simulink model "sm_ratchet_lifter"  (R2020b)
settings: Solver=daessc  StartTime=0.0  StopTime=20  MaxStep=1e-3  RelTol=1e-3  EnableMultiTasking=on
model workspace: external: MATLAB File sm_ratchet_lifter_parameters.m (data not in the file)
undefined symbols (not defined in the file or in its folder): climber, contact, cyl1, cyl10, cyl11, cyl12, cyl13, cyl14, cyl15, cyl2, cyl3, cyl4, cyl5, cyl6, cyl7, cyl8, cyl9, hook, init, LeftHorizCyl, LeftSlantCyl, load, rack, RightHorizCyl, RightSlantCyl, traveler, X, Y, Z
libraries: sm_lib x223, nesl_utility x4
(part 2 of 5)

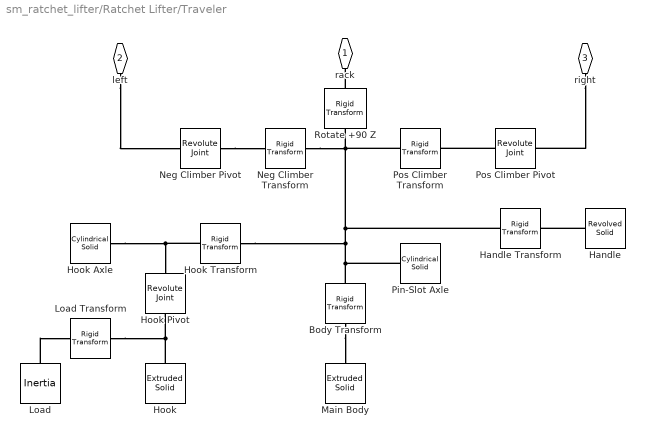
== system sm_ratchet_lifter/Ratchet Lifter/Traveler ==
  Body Transform : sm_lib/Frames and Transforms/Rigid Transform  TranslationMethod=None  TranslationStandardOffset=0  TranslationLengthUnit=m  TranslationStandardAxis=+Z  TranslationCartesianOffset=[0 0 0]  TranslationROffset=0  TranslationROffsetUnits=m  TranslationZOffset=0  TranslationZOffsetUnits=m  TranslationThetaOffset=0  TranslationThetaOffsetUnits=deg  RotationMethod=AlignedAxes  RotationAngleUnits=deg  RotationStandardAxis=+Z  RotationAngle=0.0  RotationArbitraryAxis=[0 0 1]  FollAlignAxisA=+Z  BaseAlignAxisA=+Y  FollAlignAxisB=+X  BaseAlignAxisB=-Z  RotationSequenceAxes=FollowerAxes  RotationSequence=XYX  RotationSequenceAngles=[0 0 0]  RotationSequenceAnglesUnits=deg  RotationMatrix=[1 0 0; 0 1 0; 0 0 1]
      settings: SourceProductName=Multibody
  Handle : sm_lib/Body Elements/Revolved Solid  GraphicAmbientColor=[0.15 0.15 0.15 1.0]  BasedOnType=Density  CenterOfMass=[0 0 0]  CenterOfMassUnits=m  GraphicDiffuseColor=color.handle_color  ExportConvexHullGeometry=off  Density=1000  DensityUnits=kg/m^3  DoExposeReferenceFrame=on  GraphicEmissiveColor=[0.0 0.0 0.0 1.0]  ExportEntireGeometry=off  SerializedFrames=<Frames/>  MarkerShape=Sphere  MarkerSize=10  GraphicType=FromGeometry  InertiaType=CalculateFromGeometry  Mass=1  MassUnits=kg  MomentsOfInertia=[1 1 1]  MomentsOfInertiaUnits=kg*m^2  GraphicOpacity=1.0  ProductsOfInertia=[0 0 0]  ProductsOfInertiaUnits=kg*m^2  RevolutionCrossSection=traveler.handle_xsect  RevolutionCrossSectionUnits=cm  RevolutionAngle=180  RevolutionAngleUnits=deg  RevolutionExtent=Full  GraphicShininess=75  GraphicSpecularColor=[0.5 0.5 0.5 1.0]  GraphicVisPropType=SimpleVisualProperties
      settings: SourceProductName=Multibody
  Handle Transform : sm_lib/Frames and Transforms/Rigid Transform  TranslationMethod=StandardAxis  TranslationStandardOffset=traveler.length / 2  TranslationLengthUnit=cm  TranslationStandardAxis=+X  TranslationCartesianOffset=[0 0 0]  TranslationROffset=0  TranslationROffsetUnits=m  TranslationZOffset=0  TranslationZOffsetUnits=m  TranslationThetaOffset=0  TranslationThetaOffsetUnits=deg  RotationMethod=AlignedAxes  RotationAngleUnits=deg  RotationStandardAxis=+Z  RotationAngle=0.0  RotationArbitraryAxis=[0 0 1]  FollAlignAxisA=+Z  BaseAlignAxisA=+X  FollAlignAxisB=+X  BaseAlignAxisB=+Z  RotationSequenceAxes=FollowerAxes  RotationSequence=XYX  RotationSequenceAngles=[0 0 0]  RotationSequenceAnglesUnits=deg  RotationMatrix=[1 0 0; 0 1 0; 0 0 1]
      settings: SourceProductName=Multibody
  Hook : sm_lib/Body Elements/Extruded Solid  GraphicAmbientColor=[0.15 0.15 0.15 1.0]  BasedOnType=Density  CenterOfMass=[0 0 0]  CenterOfMassUnits=m  GraphicDiffuseColor=color.hook_color  ExportConvexHullGeometry=off  ExtrusionCrossSection=hook.xsect  ExtrusionCrossSectionUnits=cm  Density=1000  DensityUnits=kg/m^3  DoExposeReferenceFrame=on  GraphicEmissiveColor=[0.0 0.0 0.0 1.0]  ExportEntireGeometry=off  ExtrusionLength=hook.thick  ExtrusionLengthUnits=cm  ExtrusionType=General  SerializedFrames=<Frames/>  MarkerShape=Sphere  MarkerSize=10  GraphicType=FromGeometry  InertiaType=CalculateFromGeometry  Mass=1  MassUnits=kg  MomentsOfInertia=[1 1 1]  MomentsOfInertiaUnits=kg*m^2  PolygonNumSides=3  GraphicOpacity=1.0  PolygonOuterRadius=1  PolygonOuterRadiusUnits=m  ProductsOfInertia=[0 0 0]  ProductsOfInertiaUnits=kg*m^2  GraphicShininess=75  GraphicSpecularColor=[0.5 0.5 0.5 1.0]  GraphicVisPropType=SimpleVisualProperties
      settings: SourceProductName=Multibody
  Hook Transform : sm_lib/Frames and Transforms/Rigid Transform  TranslationMethod=StandardAxis  TranslationStandardOffset=-traveler.length/2 + traveler.end_hole_length/2  TranslationLengthUnit=cm  TranslationStandardAxis=-X  TranslationCartesianOffset=[0 0 0]  TranslationROffset=0  TranslationROffsetUnits=m  TranslationZOffset=0  TranslationZOffsetUnits=m  TranslationThetaOffset=0  TranslationThetaOffsetUnits=deg  RotationMethod=None  RotationAngleUnits=deg  RotationStandardAxis=+Z  RotationAngle=0.0  RotationArbitraryAxis=[0 0 1]  FollAlignAxisA=+X  BaseAlignAxisA=+Y  FollAlignAxisB=+Y  BaseAlignAxisB=+Z  RotationSequenceAxes=FollowerAxes  RotationSequence=XYX  RotationSequenceAngles=[0 0 0]  RotationSequenceAnglesUnits=deg  RotationMatrix=[1 0 0; 0 1 0; 0 0 1]
      settings: SourceProductName=Multibody
  Hook Axle : sm_lib/Body Elements/Cylindrical Solid  GraphicAmbientColor=[0.15 0.15 0.15 1.0]  BasedOnType=Density  CenterOfMass=[0 0 0]  CenterOfMassUnits=m  GraphicDiffuseColor=color.traveler_axle_color  CylinderLength=traveler.axle_length  CylinderLengthUnits=cm  CylinderRadius=traveler.hook_axle_rad  CylinderRadiusUnits=cm  Density=1000  DensityUnits=kg/m^3  DoExposeReferenceFrame=on  GraphicEmissiveColor=[0.0 0.0 0.0 1.0]  ExportEntireGeometry=off  SerializedFrames=<Frames/>  MarkerShape=Sphere  MarkerSize=10  GraphicType=FromGeometry  InertiaType=CalculateFromGeometry  Mass=1  MassUnits=kg  MomentsOfInertia=[1 1 1]  MomentsOfInertiaUnits=kg*m^2  GraphicOpacity=1.0  ProductsOfInertia=[0 0 0]  ProductsOfInertiaUnits=kg*m^2  GraphicShininess=75  GraphicSpecularColor=[0.5 0.5 0.5 1.0]  GraphicVisPropType=SimpleVisualProperties
      settings: SourceProductName=Multibody
  Hook Pivot : sm_lib/Joints/Revolute Joint  JointMode=Normal  SenseConstraintForce=off  SenseConstraintForceX=off  SenseConstraintForceY=off  SenseConstraintForceZ=off  SenseConstraintTorque=off  SenseConstraintTorqueX=off  SenseConstraintTorqueY=off  SenseConstraintTorqueZ=off  SenseTotalForce=off  SenseTotalForceX=off  SenseTotalForceY=off  SenseTotalForceZ=off  SenseTotalTorque=off  SenseTotalTorqueX=off  SenseTotalTorqueY=off  SenseTotalTorqueZ=off  CompositeWrenchDir=FollowerOnBase  CompositeWrenchFrame=BaseFrame  EquilibriumPosition=0  EquilibriumPositionUnits=deg  SpringStiffness=0  SpringStiffnessUnits=N*m/deg  DampingCoefficient=0  DampingCoefficientUnits=N*m/(deg/s)  TorqueActuationMode=NoTorque  MotionActuationMode=ComputedMotion  SensePosition=off  SenseVelocity=off  SenseAcceleration=off  SenseTorqueForce=off  SenseLowerLimitTorqueForce=off  SenseUpperLimitTorqueForce=off  LowerLimitSpecify=off  LowerLimitBound=-90  LowerLimitBoundUnits=deg  LowerLimitStiffness=1e4  LowerLimitStiffnessUnits=N*m/deg  LowerLimitDamping=10  LowerLimitDampingUnits=N*m/(deg/s)  LowerLimitTransitionRegionWidth=0.1  LowerLimitTransitionRegionWidthUnits=deg  UpperLimitSpecify=off  UpperLimitBound=90  UpperLimitBoundUnits=deg  UpperLimitStiffness=1e4  UpperLimitStiffnessUnits=N*m/deg  UpperLimitDamping=10  UpperLimitDampingUnits=N*m/(deg/s)  UpperLimitTransitionRegionWidth=0.1  UpperLimitTransitionRegionWidthUnits=deg  PositionTargetSpecify=off  PositionTargetPriority=High  PositionTargetValue=0  PositionTargetValueUnits=deg  VelocityTargetSpecify=off  VelocityTargetPriority=High  VelocityTargetValue=0  VelocityTargetValueUnits=deg/s
      settings: SourceProductName=Multibody
  Load : sm_lib/Body Elements/Inertia  InertiaType=PointMass  Mass=load.mass  MassUnits=g  CenterOfMass=[0 0 0]  CenterOfMassUnits=m  MomentsOfInertia=[1 1 1]  MomentsOfInertiaUnits=kg*m^2  ProductsOfInertia=[0 0 0]  ProductsOfInertiaUnits=kg*m^2  GraphicType=None  MarkerShape=Inertia  MarkerSize=20  GraphicVisPropType=SimpleVisualProperties  GraphicDiffuseColor=[0.5 0.5 0.5]  GraphicSpecularColor=[0.5 0.5 0.5 1.0]  GraphicAmbientColor=[0.15 0.15 0.15 1.0]  GraphicEmissiveColor=[0.0 0.0 0.0 1.0]  GraphicShininess=75  GraphicOpacity=1.0
      settings: SourceProductName=Multibody
  Load Transform : sm_lib/Frames and Transforms/Rigid Transform  TranslationMethod=Cartesian  TranslationStandardOffset=0  TranslationLengthUnit=cm  TranslationStandardAxis=+Z  TranslationCartesianOffset=[hook.offset, 0] + load.dist * [0 -1 0]  TranslationROffset=0  TranslationROffsetUnits=m  TranslationZOffset=0  TranslationZOffsetUnits=m  TranslationThetaOffset=0  TranslationThetaOffsetUnits=deg  RotationMethod=None  RotationAngleUnits=deg  RotationStandardAxis=+Z  RotationAngle=0.0  RotationArbitraryAxis=[0 0 1]  FollAlignAxisA=+X  BaseAlignAxisA=+Y  FollAlignAxisB=+Y  BaseAlignAxisB=+Z  RotationSequenceAxes=FollowerAxes  RotationSequence=XYX  RotationSequenceAngles=[0 0 0]  RotationSequenceAnglesUnits=deg  RotationMatrix=[1 0 0; 0 1 0; 0 0 1]
      settings: SourceProductName=Multibody
  Main Body : sm_lib/Body Elements/Extruded Solid  GraphicAmbientColor=[0.15 0.15 0.15 1.0]  BasedOnType=Density  CenterOfMass=[0 0 0]  CenterOfMassUnits=m  GraphicDiffuseColor=color.traveler_color  ExportConvexHullGeometry=off  ExtrusionCrossSection=traveler.xsect  ExtrusionCrossSectionUnits=cm  Density=1000  DensityUnits=kg/m^3  DoExposeReferenceFrame=on  GraphicEmissiveColor=[0.0 0.0 0.0 1.0]  ExportEntireGeometry=off  ExtrusionLength=traveler.width  ExtrusionLengthUnits=cm  ExtrusionType=General  SerializedFrames=<Frames/>  MarkerShape=Sphere  MarkerSize=10  GraphicType=FromGeometry  InertiaType=CalculateFromGeometry  Mass=1  MassUnits=kg  MomentsOfInertia=[1 1 1]  MomentsOfInertiaUnits=kg*m^2  PolygonNumSides=3  GraphicOpacity=1.0  PolygonOuterRadius=1  PolygonOuterRadiusUnits=m  ProductsOfInertia=[0 0 0]  ProductsOfInertiaUnits=kg*m^2  GraphicShininess=75  GraphicSpecularColor=[0.5 0.5 0.5 1.0]  GraphicVisPropType=SimpleVisualProperties
      settings: SourceProductName=Multibody
  Neg Climber Pivot : sm_lib/Joints/Revolute Joint  JointMode=Normal  SenseConstraintForce=off  SenseConstraintForceX=off  SenseConstraintForceY=off  SenseConstraintForceZ=off  SenseConstraintTorque=off  SenseConstraintTorqueX=off  SenseConstraintTorqueY=off  SenseConstraintTorqueZ=off  SenseTotalForce=off  SenseTotalForceX=off  SenseTotalForceY=off  SenseTotalForceZ=off  SenseTotalTorque=off  SenseTotalTorqueX=off  SenseTotalTorqueY=off  SenseTotalTorqueZ=off  CompositeWrenchDir=FollowerOnBase  CompositeWrenchFrame=BaseFrame  EquilibriumPosition=0  EquilibriumPositionUnits=deg  SpringStiffness=0  SpringStiffnessUnits=N*m/deg  DampingCoefficient=0  DampingCoefficientUnits=N*m/(deg/s)  TorqueActuationMode=NoTorque  MotionActuationMode=ComputedMotion  SensePosition=off  SenseVelocity=off  SenseAcceleration=off  SenseTorqueForce=off  SenseLowerLimitTorqueForce=off  SenseUpperLimitTorqueForce=off  LowerLimitSpecify=off  LowerLimitBound=-90  LowerLimitBoundUnits=deg  LowerLimitStiffness=1e4  LowerLimitStiffnessUnits=N*m/deg  LowerLimitDamping=10  LowerLimitDampingUnits=N*m/(deg/s)  LowerLimitTransitionRegionWidth=0.1  LowerLimitTransitionRegionWidthUnits=deg  UpperLimitSpecify=off  UpperLimitBound=90  UpperLimitBoundUnits=deg  UpperLimitStiffness=1e4  UpperLimitStiffnessUnits=N*m/deg  UpperLimitDamping=10  UpperLimitDampingUnits=N*m/(deg/s)  UpperLimitTransitionRegionWidth=0.1  UpperLimitTransitionRegionWidthUnits=deg  PositionTargetSpecify=on  PositionTargetPriority=High  PositionTargetValue=pi/2 + init.climber_angle  PositionTargetValueUnits=rad  VelocityTargetSpecify=off  VelocityTargetPriority=High  VelocityTargetValue=0  VelocityTargetValueUnits=deg/s
      settings: SourceProductName=Multibody
  Neg Climber Transform : sm_lib/Frames and Transforms/Rigid Transform  TranslationMethod=StandardAxis  TranslationStandardOffset=traveler.climber_offset  TranslationLengthUnit=cm  TranslationStandardAxis=-X  TranslationCartesianOffset=[0 0 0]  TranslationROffset=0  TranslationROffsetUnits=m  TranslationZOffset=0  TranslationZOffsetUnits=m  TranslationThetaOffset=0  TranslationThetaOffsetUnits=deg  RotationMethod=None  RotationAngleUnits=deg  RotationStandardAxis=+Z  RotationAngle=0.0  RotationArbitraryAxis=[0 0 1]  FollAlignAxisA=+X  BaseAlignAxisA=+Y  FollAlignAxisB=+Y  BaseAlignAxisB=+Z  RotationSequenceAxes=FollowerAxes  RotationSequence=XYX  RotationSequenceAngles=[0 0 0]  RotationSequenceAnglesUnits=deg  RotationMatrix=[1 0 0; 0 1 0; 0 0 1]
      settings: SourceProductName=Multibody
  Pin-Slot Axle : sm_lib/Body Elements/Cylindrical Solid  GraphicAmbientColor=[0.15 0.15 0.15 1.0]  BasedOnType=Density  CenterOfMass=[0 0 0]  CenterOfMassUnits=m  GraphicDiffuseColor=color.traveler_axle_color  CylinderLength=traveler.axle_length  CylinderLengthUnits=cm  CylinderRadius=traveler.slot_half_width  CylinderRadiusUnits=cm  Density=1000  DensityUnits=kg/m^3  DoExposeReferenceFrame=on  GraphicEmissiveColor=[0.0 0.0 0.0 1.0]  ExportEntireGeometry=off  SerializedFrames=<Frames/>  MarkerShape=Sphere  MarkerSize=10  GraphicType=FromGeometry  InertiaType=CalculateFromGeometry  Mass=1  MassUnits=kg  MomentsOfInertia=[1 1 1]  MomentsOfInertiaUnits=kg*m^2  GraphicOpacity=1.0  ProductsOfInertia=[0 0 0]  ProductsOfInertiaUnits=kg*m^2  GraphicShininess=75  GraphicSpecularColor=[0.5 0.5 0.5 1.0]  GraphicVisPropType=SimpleVisualProperties
      settings: SourceProductName=Multibody
  Pos Climber Pivot : sm_lib/Joints/Revolute Joint  JointMode=Normal  SenseConstraintForce=off  SenseConstraintForceX=off  SenseConstraintForceY=off  SenseConstraintForceZ=off  SenseConstraintTorque=off  SenseConstraintTorqueX=off  SenseConstraintTorqueY=off  SenseConstraintTorqueZ=off  SenseTotalForce=off  SenseTotalForceX=off  SenseTotalForceY=off  SenseTotalForceZ=off  SenseTotalTorque=off  SenseTotalTorqueX=off  SenseTotalTorqueY=off  SenseTotalTorqueZ=off  CompositeWrenchDir=FollowerOnBase  CompositeWrenchFrame=BaseFrame  EquilibriumPosition=0  EquilibriumPositionUnits=deg  SpringStiffness=0  SpringStiffnessUnits=N*m/deg  DampingCoefficient=0  DampingCoefficientUnits=N*m/(deg/s)  TorqueActuationMode=NoTorque  MotionActuationMode=ComputedMotion  SensePosition=off  SenseVelocity=off  SenseAcceleration=off  SenseTorqueForce=off  SenseLowerLimitTorqueForce=off  SenseUpperLimitTorqueForce=off  LowerLimitSpecify=off  LowerLimitBound=-90  LowerLimitBoundUnits=deg  LowerLimitStiffness=1e4  LowerLimitStiffnessUnits=N*m/deg  LowerLimitDamping=10  LowerLimitDampingUnits=N*m/(deg/s)  LowerLimitTransitionRegionWidth=0.1  LowerLimitTransitionRegionWidthUnits=deg  UpperLimitSpecify=off  UpperLimitBound=90  UpperLimitBoundUnits=deg  UpperLimitStiffness=1e4  UpperLimitStiffnessUnits=N*m/deg  UpperLimitDamping=10  UpperLimitDampingUnits=N*m/(deg/s)  UpperLimitTransitionRegionWidth=0.1  UpperLimitTransitionRegionWidthUnits=deg  PositionTargetSpecify=on  PositionTargetPriority=High  PositionTargetValue=pi/2 - init.climber_angle  PositionTargetValueUnits=rad  VelocityTargetSpecify=off  VelocityTargetPriority=High  VelocityTargetValue=0  VelocityTargetValueUnits=deg/s
      settings: SourceProductName=Multibody
  Pos Climber Transform : sm_lib/Frames and Transforms/Rigid Transform  TranslationMethod=StandardAxis  TranslationStandardOffset=traveler.climber_offset  TranslationLengthUnit=cm  TranslationStandardAxis=+X  TranslationCartesianOffset=[0 0 0]  TranslationROffset=0  TranslationROffsetUnits=m  TranslationZOffset=0  TranslationZOffsetUnits=m  TranslationThetaOffset=0  TranslationThetaOffsetUnits=deg  RotationMethod=None  RotationAngleUnits=deg  RotationStandardAxis=+Z  RotationAngle=0.0  RotationArbitraryAxis=[0 0 1]  FollAlignAxisA=+X  BaseAlignAxisA=+Y  FollAlignAxisB=+Y  BaseAlignAxisB=+Z  RotationSequenceAxes=FollowerAxes  RotationSequence=XYX  RotationSequenceAngles=[0 0 0]  RotationSequenceAnglesUnits=deg  RotationMatrix=[1 0 0; 0 1 0; 0 0 1]
      settings: SourceProductName=Multibody
  Rotate +90 Z : sm_lib/Frames and Transforms/Rigid Transform  TranslationMethod=None  TranslationStandardOffset=0  TranslationLengthUnit=m  TranslationStandardAxis=+Z  TranslationCartesianOffset=[0 0 0]  TranslationROffset=0  TranslationROffsetUnits=m  TranslationZOffset=0  TranslationZOffsetUnits=m  TranslationThetaOffset=0  TranslationThetaOffsetUnits=deg  RotationMethod=StandardAxis  RotationAngleUnits=deg  RotationStandardAxis=+Z  RotationAngle=90  RotationArbitraryAxis=[0 0 1]  FollAlignAxisA=+X  BaseAlignAxisA=+Y  FollAlignAxisB=+Y  BaseAlignAxisB=+Z  RotationSequenceAxes=FollowerAxes  RotationSequence=XYX  RotationSequenceAngles=[0 0 0]  RotationSequenceAnglesUnits=deg  RotationMatrix=[1 0 0; 0 1 0; 0 0 1]
      settings: SourceProductName=Multibody
  rack : PMIOPort  Side=Left
  left : PMIOPort  Port=2  Side=Left
  right : PMIOPort  Port=3  Side=Right
  connections:
  Pin-Slot Axle/RConn1 -- Hook Transform/RConn1 -- Handle Transform/LConn1 -- Pos Climber Transform/LConn1 -- Rotate +90 Z/LConn1 -- Neg Climber Transform/LConn1 -- Body Transform/LConn1
  Pos Climber Pivot/LConn1 -- Pos Climber Transform/RConn1
  left/RConn1 -- Neg Climber Pivot/RConn1
  right/RConn1 -- Pos Climber Pivot/RConn1
  Rotate +90 Z/RConn1 -- rack/RConn1
  Neg Climber Pivot/LConn1 -- Neg Climber Transform/RConn1
  Handle/RConn1 -- Handle Transform/RConn1
  Body Transform/RConn1 -- Main Body/RConn1
  Hook Transform/LConn1 -- Hook Axle/RConn1 -- Hook Pivot/LConn1
  Hook/RConn1 -- Load Transform/LConn1 -- Hook Pivot/RConn1
  Load/RConn1 -- Load Transform/RConn1

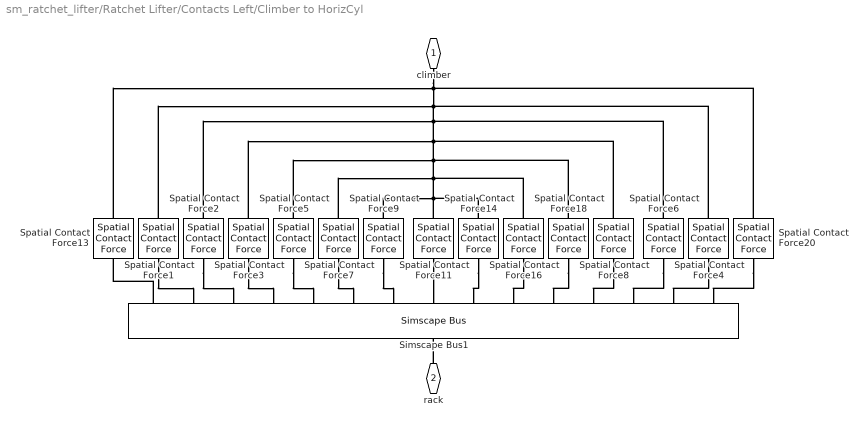
== system sm_ratchet_lifter/Ratchet Lifter/Contacts Left/Climber to HorizCyl ==
  Simscape Bus1 : SimscapeBus  HierarchyStrings=cyl15;cyl14;cyl13;cyl12;cyl11;cyl10;cyl9;cyl8;cyl7;cyl6;cyl5;cyl4;cyl3;cyl2;cyl1
  Spatial Contact Force{1..9,11,13..14,16,18,20} (15 alike) : sm_lib/Forces and Torques/Spatial Contact Force  CoefficientOfDynamicFriction=muk  CoefficientOfStaticFriction=mus  NormalDamping=b  NormalDampingUnits=N/(m/s)  NormalStiffness=k  NormalStiffnessUnits=N/m  FrictionalCriticalVelocity=cv  FrictionalCriticalVelocityUnits=cm/s  ZeroCrossDetectContactStartAndEnd=off  SenseFrictionalForceMagnitude=off  SenseNormalForceMagnitude=off  SenseSeparationDistance=off  NormalTransitionRegionWidth=tau  NormalTransitionRegionWidthUnits=mm  FrictionType=SmoothStickSlip
      settings: SourceProductName=Multibody
  climber : PMIOPort  Side=Right
  rack : PMIOPort  Port=2  Side=Left
  connections:
  Spatial Contact Force13/RConn1 -- Spatial Contact Force20/RConn1 -- Spatial Contact Force4/RConn1 -- Spatial Contact Force1/RConn1 -- Spatial Contact Force6/RConn1 -- Spatial Contact Force2/RConn1 -- Spatial Contact Force8/RConn1 -- Spatial Contact Force3/RConn1 -- Spatial Contact Force18/RConn1 -- Spatial Contact Force5/RConn1 -- Spatial Contact Force16/RConn1 -- Spatial Contact Force7/RConn1 -- Spatial Contact Force14/RConn1 -- Spatial Contact Force11/RConn1 -- Spatial Contact Force9/RConn1 -- climber/RConn1
  Spatial Contact Force11/LConn1 -- Simscape Bus1/LConn8
  Spatial Contact Force8/LConn1 -- Simscape Bus1/LConn12
  Spatial Contact Force7/LConn1 -- Simscape Bus1/LConn6
  Simscape Bus1/LConn1 -- Spatial Contact Force13/LConn1
  Spatial Contact Force5/LConn1 -- Simscape Bus1/LConn5
  Spatial Contact Force2/LConn1 -- Simscape Bus1/LConn3
  Spatial Contact Force18/LConn1 -- Simscape Bus1/LConn11
  Spatial Contact Force9/LConn1 -- Simscape Bus1/LConn7
  Spatial Contact Force14/LConn1 -- Simscape Bus1/LConn9
  Spatial Contact Force1/LConn1 -- Simscape Bus1/LConn2
  rack/RConn1 -- Simscape Bus1/RConn1
  Spatial Contact Force16/LConn1 -- Simscape Bus1/LConn10
  Spatial Contact Force20/LConn1 -- Simscape Bus1/LConn15
  Spatial Contact Force4/LConn1 -- Simscape Bus1/LConn14
  Spatial Contact Force3/LConn1 -- Simscape Bus1/LConn4
  Spatial Contact Force6/LConn1 -- Simscape Bus1/LConn13

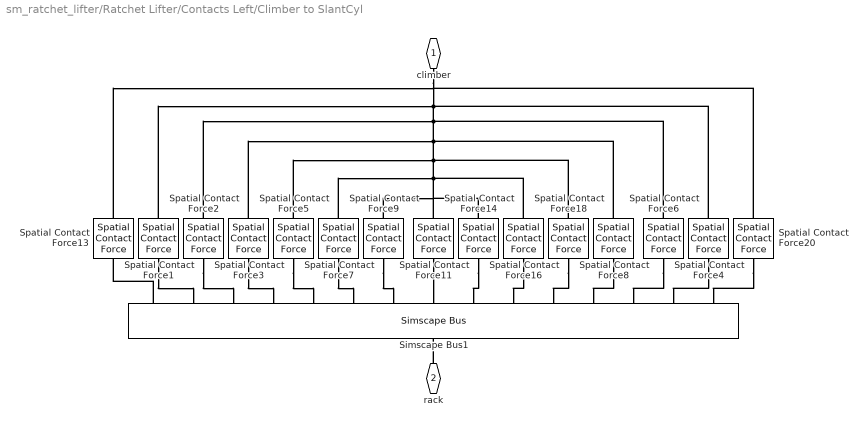
== system sm_ratchet_lifter/Ratchet Lifter/Contacts Left/Climber to SlantCyl ==
  Simscape Bus1 : SimscapeBus  HierarchyStrings=cyl15;cyl14;cyl13;cyl12;cyl11;cyl10;cyl9;cyl8;cyl7;cyl6;cyl5;cyl4;cyl3;cyl2;cyl1
  Spatial Contact Force{1..9,11,13..14,16,18,20} (15 alike) : sm_lib/Forces and Torques/Spatial Contact Force  CoefficientOfDynamicFriction=muk  CoefficientOfStaticFriction=mus  NormalDamping=b  NormalDampingUnits=N/(m/s)  NormalStiffness=k  NormalStiffnessUnits=N/m  FrictionalCriticalVelocity=cv  FrictionalCriticalVelocityUnits=cm/s  ZeroCrossDetectContactStartAndEnd=off  SenseFrictionalForceMagnitude=off  SenseNormalForceMagnitude=off  SenseSeparationDistance=off  NormalTransitionRegionWidth=tau  NormalTransitionRegionWidthUnits=mm  FrictionType=SmoothStickSlip
      settings: SourceProductName=Multibody
  climber : PMIOPort  Side=Right
  rack : PMIOPort  Port=2  Side=Left
  connections:
  Spatial Contact Force14/RConn1 -- Spatial Contact Force11/RConn1 -- Spatial Contact Force9/RConn1 -- Spatial Contact Force16/RConn1 -- Spatial Contact Force7/RConn1 -- Spatial Contact Force18/RConn1 -- Spatial Contact Force5/RConn1 -- Spatial Contact Force8/RConn1 -- Spatial Contact Force3/RConn1 -- Spatial Contact Force6/RConn1 -- Spatial Contact Force2/RConn1 -- Spatial Contact Force4/RConn1 -- Spatial Contact Force1/RConn1 -- Spatial Contact Force20/RConn1 -- climber/RConn1 -- Spatial Contact Force13/RConn1
  rack/RConn1 -- Simscape Bus1/RConn1
  Spatial Contact Force20/LConn1 -- Simscape Bus1/LConn15
  Spatial Contact Force4/LConn1 -- Simscape Bus1/LConn14
  Spatial Contact Force6/LConn1 -- Simscape Bus1/LConn13
  Spatial Contact Force8/LConn1 -- Simscape Bus1/LConn12
  Spatial Contact Force18/LConn1 -- Simscape Bus1/LConn11
  Spatial Contact Force16/LConn1 -- Simscape Bus1/LConn10
  Spatial Contact Force14/LConn1 -- Simscape Bus1/LConn9
  Spatial Contact Force11/LConn1 -- Simscape Bus1/LConn8
  Spatial Contact Force9/LConn1 -- Simscape Bus1/LConn7
  Spatial Contact Force7/LConn1 -- Simscape Bus1/LConn6
  Spatial Contact Force5/LConn1 -- Simscape Bus1/LConn5
  Spatial Contact Force3/LConn1 -- Simscape Bus1/LConn4
  Spatial Contact Force2/LConn1 -- Simscape Bus1/LConn3
  Spatial Contact Force1/LConn1 -- Simscape Bus1/LConn2
  Simscape Bus1/LConn1 -- Spatial Contact Force13/LConn1

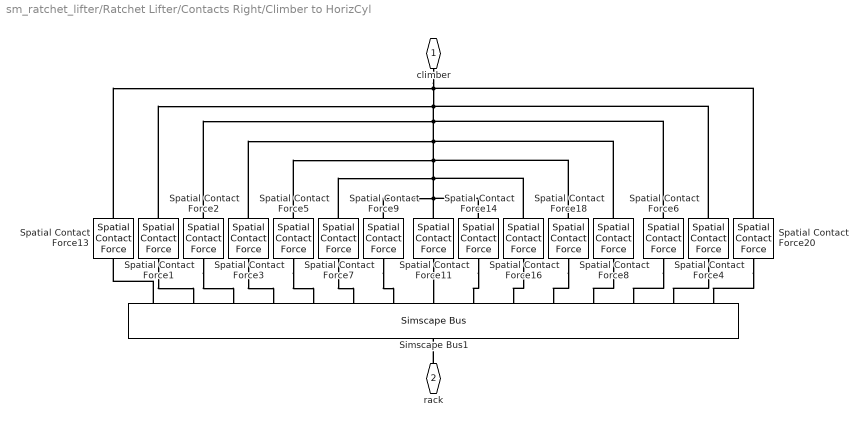
== system sm_ratchet_lifter/Ratchet Lifter/Contacts Right/Climber to HorizCyl ==
  Simscape Bus1 : SimscapeBus  HierarchyStrings=cyl15;cyl14;cyl13;cyl12;cyl11;cyl10;cyl9;cyl8;cyl7;cyl6;cyl5;cyl4;cyl3;cyl2;cyl1
  Spatial Contact Force{1..9,11,13..14,16,18,20} (15 alike) : sm_lib/Forces and Torques/Spatial Contact Force  CoefficientOfDynamicFriction=muk  CoefficientOfStaticFriction=mus  NormalDamping=b  NormalDampingUnits=N/(m/s)  NormalStiffness=k  NormalStiffnessUnits=N/m  FrictionalCriticalVelocity=cv  FrictionalCriticalVelocityUnits=cm/s  ZeroCrossDetectContactStartAndEnd=off  SenseFrictionalForceMagnitude=off  SenseNormalForceMagnitude=off  SenseSeparationDistance=off  NormalTransitionRegionWidth=tau  NormalTransitionRegionWidthUnits=mm  FrictionType=SmoothStickSlip
      settings: SourceProductName=Multibody
  climber : PMIOPort  Side=Right
  rack : PMIOPort  Port=2  Side=Left
  connections:
  Spatial Contact Force13/RConn1 -- Spatial Contact Force20/RConn1 -- Spatial Contact Force4/RConn1 -- Spatial Contact Force1/RConn1 -- Spatial Contact Force6/RConn1 -- Spatial Contact Force2/RConn1 -- Spatial Contact Force8/RConn1 -- Spatial Contact Force3/RConn1 -- Spatial Contact Force18/RConn1 -- Spatial Contact Force5/RConn1 -- Spatial Contact Force16/RConn1 -- Spatial Contact Force7/RConn1 -- Spatial Contact Force14/RConn1 -- Spatial Contact Force11/RConn1 -- Spatial Contact Force9/RConn1 -- climber/RConn1
  Spatial Contact Force11/LConn1 -- Simscape Bus1/LConn8
  Spatial Contact Force8/LConn1 -- Simscape Bus1/LConn12
  Spatial Contact Force7/LConn1 -- Simscape Bus1/LConn6
  Simscape Bus1/LConn1 -- Spatial Contact Force13/LConn1
  Spatial Contact Force5/LConn1 -- Simscape Bus1/LConn5
  Spatial Contact Force2/LConn1 -- Simscape Bus1/LConn3
  Spatial Contact Force18/LConn1 -- Simscape Bus1/LConn11
  Spatial Contact Force9/LConn1 -- Simscape Bus1/LConn7
  Spatial Contact Force14/LConn1 -- Simscape Bus1/LConn9
  Spatial Contact Force1/LConn1 -- Simscape Bus1/LConn2
  rack/RConn1 -- Simscape Bus1/RConn1
  Spatial Contact Force16/LConn1 -- Simscape Bus1/LConn10
  Spatial Contact Force20/LConn1 -- Simscape Bus1/LConn15
  Spatial Contact Force4/LConn1 -- Simscape Bus1/LConn14
  Spatial Contact Force3/LConn1 -- Simscape Bus1/LConn4
  Spatial Contact Force6/LConn1 -- Simscape Bus1/LConn13

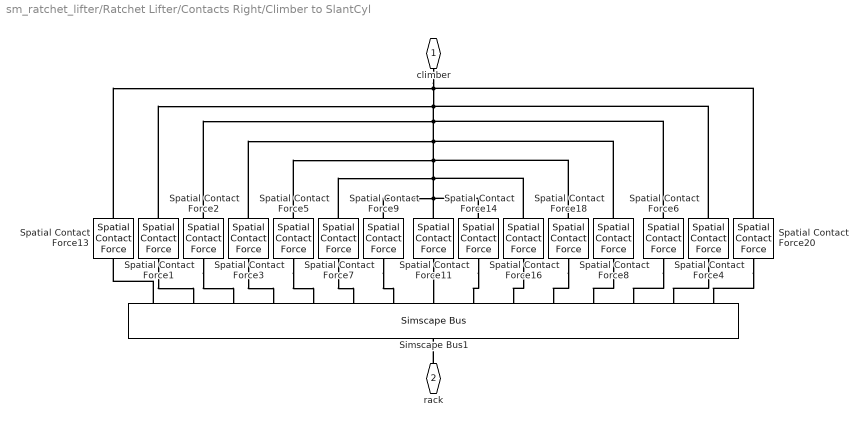
== system sm_ratchet_lifter/Ratchet Lifter/Contacts Right/Climber to SlantCyl ==
  Simscape Bus1 : SimscapeBus  HierarchyStrings=cyl15;cyl14;cyl13;cyl12;cyl11;cyl10;cyl9;cyl8;cyl7;cyl6;cyl5;cyl4;cyl3;cyl2;cyl1
  Spatial Contact Force{1..9,11,13..14,16,18,20} (15 alike) : sm_lib/Forces and Torques/Spatial Contact Force  CoefficientOfDynamicFriction=muk  CoefficientOfStaticFriction=mus  NormalDamping=b  NormalDampingUnits=N/(m/s)  NormalStiffness=k  NormalStiffnessUnits=N/m  FrictionalCriticalVelocity=cv  FrictionalCriticalVelocityUnits=cm/s  ZeroCrossDetectContactStartAndEnd=off  SenseFrictionalForceMagnitude=off  SenseNormalForceMagnitude=off  SenseSeparationDistance=off  NormalTransitionRegionWidth=tau  NormalTransitionRegionWidthUnits=mm  FrictionType=SmoothStickSlip
      settings: SourceProductName=Multibody
  climber : PMIOPort  Side=Right
  rack : PMIOPort  Port=2  Side=Left
  connections:
  Spatial Contact Force13/RConn1 -- Spatial Contact Force20/RConn1 -- Spatial Contact Force4/RConn1 -- Spatial Contact Force1/RConn1 -- Spatial Contact Force6/RConn1 -- Spatial Contact Force2/RConn1 -- Spatial Contact Force8/RConn1 -- Spatial Contact Force3/RConn1 -- Spatial Contact Force18/RConn1 -- Spatial Contact Force5/RConn1 -- Spatial Contact Force16/RConn1 -- Spatial Contact Force7/RConn1 -- Spatial Contact Force14/RConn1 -- Spatial Contact Force11/RConn1 -- Spatial Contact Force9/RConn1 -- climber/RConn1
  Spatial Contact Force11/LConn1 -- Simscape Bus1/LConn8
  Spatial Contact Force8/LConn1 -- Simscape Bus1/LConn12
  Spatial Contact Force7/LConn1 -- Simscape Bus1/LConn6
  Simscape Bus1/LConn1 -- Spatial Contact Force13/LConn1
  Spatial Contact Force5/LConn1 -- Simscape Bus1/LConn5
  Spatial Contact Force2/LConn1 -- Simscape Bus1/LConn3
  Spatial Contact Force18/LConn1 -- Simscape Bus1/LConn11
  Spatial Contact Force9/LConn1 -- Simscape Bus1/LConn7
  Spatial Contact Force14/LConn1 -- Simscape Bus1/LConn9
  Spatial Contact Force1/LConn1 -- Simscape Bus1/LConn2
  rack/RConn1 -- Simscape Bus1/RConn1
  Spatial Contact Force16/LConn1 -- Simscape Bus1/LConn10
  Spatial Contact Force20/LConn1 -- Simscape Bus1/LConn15
  Spatial Contact Force4/LConn1 -- Simscape Bus1/LConn14
  Spatial Contact Force3/LConn1 -- Simscape Bus1/LConn4
  Spatial Contact Force6/LConn1 -- Simscape Bus1/LConn13

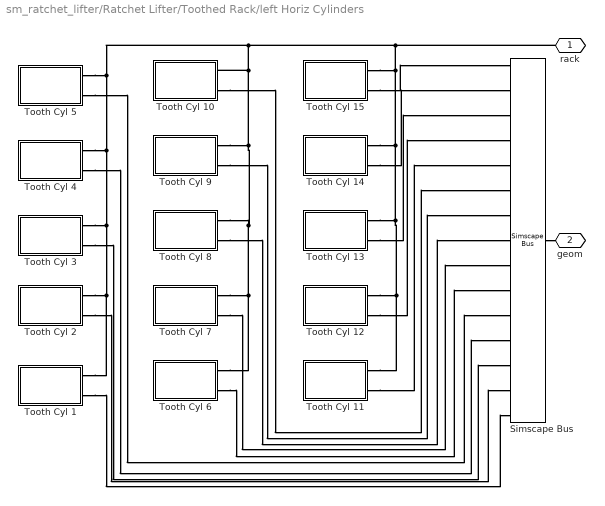
== system sm_ratchet_lifter/Ratchet Lifter/Toothed Rack/left Horiz Cylinders ==
  Simscape Bus : SimscapeBus  HierarchyStrings=cyl15;cyl14;cyl13;cyl12;cyl11;cyl10;cyl9;cyl8;cyl7;cyl6;cyl5;cyl4;cyl3;cyl2;cyl1
  Tooth Cyl 1 : Subsystem  mask{idx=1}
      mask prompts: idx "Index"
  Tooth Cyl 10 : Subsystem  mask{idx=10}
      mask prompts: idx "Index"
  Tooth Cyl 11 : Subsystem  mask{idx=11}
      mask prompts: idx "Index"
  Tooth Cyl 12 : Subsystem  mask{idx=12}
      mask prompts: idx "Index"
  Tooth Cyl 13 : Subsystem  mask{idx=13}
      mask prompts: idx "Index"
  Tooth Cyl 14 : Subsystem  mask{idx=14}
      mask prompts: idx "Index"
  Tooth Cyl 15 : Subsystem  mask{idx=15}
      mask prompts: idx "Index"
  Tooth Cyl 2 : Subsystem  mask{idx=2}
      mask prompts: idx "Index"
  Tooth Cyl 3 : Subsystem  mask{idx=3}
      mask prompts: idx "Index"
  Tooth Cyl 4 : Subsystem  mask{idx=4}
      mask prompts: idx "Index"
  Tooth Cyl 5 : Subsystem  mask{idx=5}
      mask prompts: idx "Index"
  Tooth Cyl 6 : Subsystem  mask{idx=6}
      mask prompts: idx "Index"
  Tooth Cyl 7 : Subsystem  mask{idx=7}
      mask prompts: idx "Index"
  Tooth Cyl 8 : Subsystem  mask{idx=8}
      mask prompts: idx "Index"
  Tooth Cyl 9 : Subsystem  mask{idx=9}
      mask prompts: idx "Index"
  rack : PMIOPort  Side=Left
  geom : PMIOPort  Port=2  Side=Right
  connections:
  Tooth Cyl 11/RConn1 -- Tooth Cyl 12/RConn1 -- Tooth Cyl 13/RConn1 -- Tooth Cyl 14/RConn1 -- Tooth Cyl 15/RConn1 -- rack/RConn1 -- Tooth Cyl 8/RConn1 -- Tooth Cyl 6/RConn1 -- Tooth Cyl 7/RConn1 -- Tooth Cyl 9/RConn1 -- Tooth Cyl 10/RConn1 -- Tooth Cyl 4/RConn1 -- Tooth Cyl 3/RConn1 -- Tooth Cyl 1/RConn1 -- Tooth Cyl 2/RConn1 -- Tooth Cyl 5/RConn1
  Tooth Cyl 14/RConn2 -- Simscape Bus/LConn2
  Tooth Cyl 4/RConn2 -- Simscape Bus/LConn12
  Tooth Cyl 7/RConn2 -- Simscape Bus/LConn9
  Tooth Cyl 11/RConn2 -- Simscape Bus/LConn5
  Tooth Cyl 8/RConn2 -- Simscape Bus/LConn8
  Tooth Cyl 10/RConn2 -- Simscape Bus/LConn6
  Tooth Cyl 9/RConn2 -- Simscape Bus/LConn7
  Tooth Cyl 6/RConn2 -- Simscape Bus/LConn10
  Tooth Cyl 5/RConn2 -- Simscape Bus/LConn11
  Tooth Cyl 12/RConn2 -- Simscape Bus/LConn4
  Tooth Cyl 2/RConn2 -- Simscape Bus/LConn14
  Tooth Cyl 1/RConn2 -- Simscape Bus/LConn15
  Tooth Cyl 13/RConn2 -- Simscape Bus/LConn3
  Tooth Cyl 15/RConn2 -- Simscape Bus/LConn1
  Tooth Cyl 3/RConn2 -- Simscape Bus/LConn13
  Simscape Bus/RConn1 -- geom/RConn1

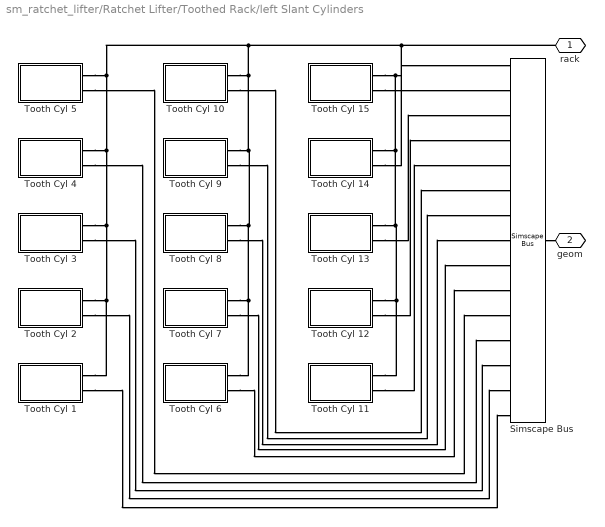
== system sm_ratchet_lifter/Ratchet Lifter/Toothed Rack/left Slant Cylinders ==
  Simscape Bus : SimscapeBus  HierarchyStrings=cyl15;cyl14;cyl13;cyl12;cyl11;cyl10;cyl9;cyl8;cyl7;cyl6;cyl5;cyl4;cyl3;cyl2;cyl1
  Tooth Cyl 1 : Subsystem  mask{idx=1}
      mask prompts: idx "Index"
  Tooth Cyl 10 : Subsystem  mask{idx=10}
      mask prompts: idx "Index"
  Tooth Cyl 11 : Subsystem  mask{idx=11}
      mask prompts: idx "Index"
  Tooth Cyl 12 : Subsystem  mask{idx=12}
      mask prompts: idx "Index"
  Tooth Cyl 13 : Subsystem  mask{idx=13}
      mask prompts: idx "Index"
  Tooth Cyl 14 : Subsystem  mask{idx=14}
      mask prompts: idx "Index"
  Tooth Cyl 15 : Subsystem  mask{idx=15}
      mask prompts: idx "Index"
  Tooth Cyl 2 : Subsystem  mask{idx=2}
      mask prompts: idx "Index"
  Tooth Cyl 3 : Subsystem  mask{idx=3}
      mask prompts: idx "Index"
  Tooth Cyl 4 : Subsystem  mask{idx=4}
      mask prompts: idx "Index"
  Tooth Cyl 5 : Subsystem  mask{idx=5}
      mask prompts: idx "Index"
  Tooth Cyl 6 : Subsystem  mask{idx=6}
      mask prompts: idx "Index"
  Tooth Cyl 7 : Subsystem  mask{idx=7}
      mask prompts: idx "Index"
  Tooth Cyl 8 : Subsystem  mask{idx=8}
      mask prompts: idx "Index"
  Tooth Cyl 9 : Subsystem  mask{idx=9}
      mask prompts: idx "Index"
  rack : PMIOPort  Side=Left
  geom : PMIOPort  Port=2  Side=Right
  connections:
  Tooth Cyl 11/RConn1 -- Tooth Cyl 12/RConn1 -- Tooth Cyl 13/RConn1 -- Tooth Cyl 14/RConn1 -- Tooth Cyl 15/RConn1 -- rack/RConn1 -- Tooth Cyl 5/RConn1 -- Tooth Cyl 4/RConn1 -- Tooth Cyl 3/RConn1 -- Tooth Cyl 2/RConn1 -- Tooth Cyl 1/RConn1 -- Tooth Cyl 10/RConn1 -- Tooth Cyl 7/RConn1 -- Tooth Cyl 6/RConn1 -- Tooth Cyl 8/RConn1 -- Tooth Cyl 9/RConn1
  Simscape Bus/RConn1 -- geom/RConn1
  Tooth Cyl 11/RConn2 -- Simscape Bus/LConn5
  Tooth Cyl 12/RConn2 -- Simscape Bus/LConn4
  Tooth Cyl 13/RConn2 -- Simscape Bus/LConn3
  Tooth Cyl 14/RConn2 -- Simscape Bus/LConn2
  Tooth Cyl 15/RConn2 -- Simscape Bus/LConn1
  Tooth Cyl 10/RConn2 -- Simscape Bus/LConn6
  Tooth Cyl 9/RConn2 -- Simscape Bus/LConn7
  Tooth Cyl 8/RConn2 -- Simscape Bus/LConn8
  Tooth Cyl 7/RConn2 -- Simscape Bus/LConn9
  Tooth Cyl 6/RConn2 -- Simscape Bus/LConn10
  Tooth Cyl 1/RConn2 -- Simscape Bus/LConn15
  Tooth Cyl 2/RConn2 -- Simscape Bus/LConn14
  Tooth Cyl 3/RConn2 -- Simscape Bus/LConn13
  Tooth Cyl 4/RConn2 -- Simscape Bus/LConn12
  Tooth Cyl 5/RConn2 -- Simscape Bus/LConn11

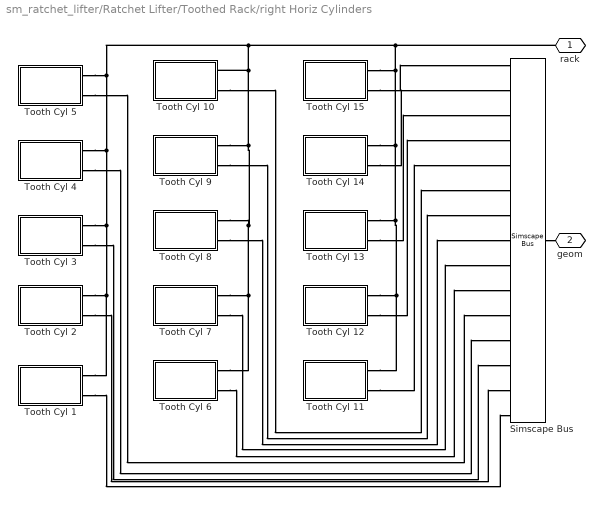
== system sm_ratchet_lifter/Ratchet Lifter/Toothed Rack/right Horiz Cylinders ==
  Simscape Bus : SimscapeBus  HierarchyStrings=cyl15;cyl14;cyl13;cyl12;cyl11;cyl10;cyl9;cyl8;cyl7;cyl6;cyl5;cyl4;cyl3;cyl2;cyl1
  Tooth Cyl 1 : Subsystem  mask{idx=1}
      mask prompts: idx "Index"
  Tooth Cyl 10 : Subsystem  mask{idx=10}
      mask prompts: idx "Index"
  Tooth Cyl 11 : Subsystem  mask{idx=11}
      mask prompts: idx "Index"
  Tooth Cyl 12 : Subsystem  mask{idx=12}
      mask prompts: idx "Index"
  Tooth Cyl 13 : Subsystem  mask{idx=13}
      mask prompts: idx "Index"
  Tooth Cyl 14 : Subsystem  mask{idx=14}
      mask prompts: idx "Index"
  Tooth Cyl 15 : Subsystem  mask{idx=15}
      mask prompts: idx "Index"
  Tooth Cyl 2 : Subsystem  mask{idx=2}
      mask prompts: idx "Index"
  Tooth Cyl 3 : Subsystem  mask{idx=3}
      mask prompts: idx "Index"
  Tooth Cyl 4 : Subsystem  mask{idx=4}
      mask prompts: idx "Index"
  Tooth Cyl 5 : Subsystem  mask{idx=5}
      mask prompts: idx "Index"
  Tooth Cyl 6 : Subsystem  mask{idx=6}
      mask prompts: idx "Index"
  Tooth Cyl 7 : Subsystem  mask{idx=7}
      mask prompts: idx "Index"
  Tooth Cyl 8 : Subsystem  mask{idx=8}
      mask prompts: idx "Index"
  Tooth Cyl 9 : Subsystem  mask{idx=9}
      mask prompts: idx "Index"
  rack : PMIOPort  Side=Left
  geom : PMIOPort  Port=2  Side=Right
  connections:
  Tooth Cyl 5/RConn1 -- Tooth Cyl 4/RConn1 -- Tooth Cyl 3/RConn1 -- Tooth Cyl 1/RConn1 -- Tooth Cyl 2/RConn1 -- Tooth Cyl 8/RConn1 -- Tooth Cyl 6/RConn1 -- Tooth Cyl 7/RConn1 -- Tooth Cyl 9/RConn1 -- Tooth Cyl 10/RConn1 -- rack/RConn1 -- Tooth Cyl 15/RConn1 -- Tooth Cyl 14/RConn1 -- Tooth Cyl 11/RConn1 -- Tooth Cyl 12/RConn1 -- Tooth Cyl 13/RConn1
  Tooth Cyl 9/RConn2 -- Simscape Bus/LConn7
  Tooth Cyl 7/RConn2 -- Simscape Bus/LConn9
  Simscape Bus/RConn1 -- geom/RConn1
  Tooth Cyl 14/RConn2 -- Simscape Bus/LConn2
  Tooth Cyl 10/RConn2 -- Simscape Bus/LConn6
  Tooth Cyl 3/RConn2 -- Simscape Bus/LConn13
  Tooth Cyl 2/RConn2 -- Simscape Bus/LConn14
  Tooth Cyl 12/RConn2 -- Simscape Bus/LConn4
  Tooth Cyl 15/RConn2 -- Simscape Bus/LConn1
  Tooth Cyl 4/RConn2 -- Simscape Bus/LConn12
  Tooth Cyl 6/RConn2 -- Simscape Bus/LConn10
  Tooth Cyl 11/RConn2 -- Simscape Bus/LConn5
  Tooth Cyl 5/RConn2 -- Simscape Bus/LConn11
  Tooth Cyl 13/RConn2 -- Simscape Bus/LConn3
  Tooth Cyl 1/RConn2 -- Simscape Bus/LConn15
  Tooth Cyl 8/RConn2 -- Simscape Bus/LConn8

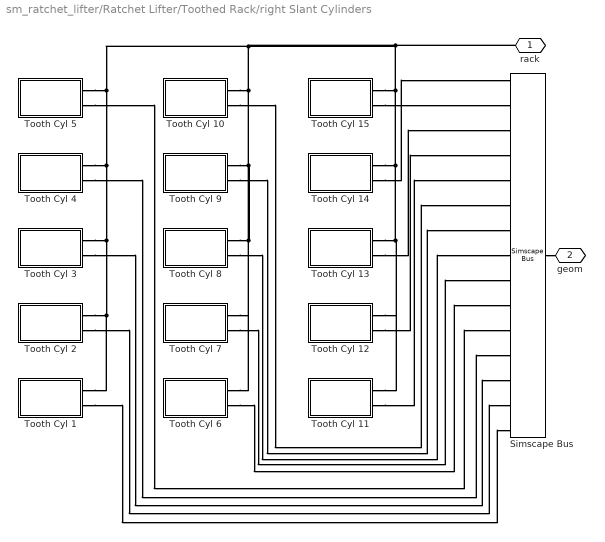
== system sm_ratchet_lifter/Ratchet Lifter/Toothed Rack/right Slant Cylinders ==
  Simscape Bus : SimscapeBus  HierarchyStrings=cyl15;cyl14;cyl13;cyl12;cyl11;cyl10;cyl9;cyl8;cyl7;cyl6;cyl5;cyl4;cyl3;cyl2;cyl1
  Tooth Cyl 1 : Subsystem  mask{idx=1}
      mask prompts: idx "Index"
  Tooth Cyl 10 : Subsystem  mask{idx=10}
      mask prompts: idx "Index"
  Tooth Cyl 11 : Subsystem  mask{idx=11}
      mask prompts: idx "Index"
  Tooth Cyl 12 : Subsystem  mask{idx=12}
      mask prompts: idx "Index"
  Tooth Cyl 13 : Subsystem  mask{idx=13}
      mask prompts: idx "Index"
  Tooth Cyl 14 : Subsystem  mask{idx=14}
      mask prompts: idx "Index"
  Tooth Cyl 15 : Subsystem  mask{idx=15}
      mask prompts: idx "Index"
  Tooth Cyl 2 : Subsystem  mask{idx=2}
      mask prompts: idx "Index"
  Tooth Cyl 3 : Subsystem  mask{idx=3}
      mask prompts: idx "Index"
  Tooth Cyl 4 : Subsystem  mask{idx=4}
      mask prompts: idx "Index"
  Tooth Cyl 5 : Subsystem  mask{idx=5}
      mask prompts: idx "Index"
  Tooth Cyl 6 : Subsystem  mask{idx=6}
      mask prompts: idx "Index"
  Tooth Cyl 7 : Subsystem  mask{idx=7}
      mask prompts: idx "Index"
  Tooth Cyl 8 : Subsystem  mask{idx=8}
      mask prompts: idx "Index"
  Tooth Cyl 9 : Subsystem  mask{idx=9}
      mask prompts: idx "Index"
  rack : PMIOPort  Side=Left
  geom : PMIOPort  Port=2  Side=Right
  connections:
  Tooth Cyl 9/RConn1 -- Tooth Cyl 10/RConn1 -- rack/RConn1 -- Tooth Cyl 15/RConn1 -- Tooth Cyl 11/RConn1 -- Tooth Cyl 12/RConn1 -- Tooth Cyl 13/RConn1 -- Tooth Cyl 14/RConn1 -- Tooth Cyl 5/RConn1 -- Tooth Cyl 4/RConn1 -- Tooth Cyl 3/RConn1 -- Tooth Cyl 2/RConn1 -- Tooth Cyl 1/RConn1 -- Tooth Cyl 7/RConn1 -- Tooth Cyl 6/RConn1 -- Tooth Cyl 8/RConn1
  Simscape Bus/RConn1 -- geom/RConn1
  Tooth Cyl 11/RConn2 -- Simscape Bus/LConn5
  Tooth Cyl 12/RConn2 -- Simscape Bus/LConn4
  Tooth Cyl 13/RConn2 -- Simscape Bus/LConn3
  Tooth Cyl 14/RConn2 -- Simscape Bus/LConn2
  Tooth Cyl 15/RConn2 -- Simscape Bus/LConn1
  Tooth Cyl 10/RConn2 -- Simscape Bus/LConn6
  Tooth Cyl 9/RConn2 -- Simscape Bus/LConn7
  Tooth Cyl 8/RConn2 -- Simscape Bus/LConn8
  Tooth Cyl 7/RConn2 -- Simscape Bus/LConn9
  Tooth Cyl 6/RConn2 -- Simscape Bus/LConn10
  Tooth Cyl 1/RConn2 -- Simscape Bus/LConn15
  Tooth Cyl 2/RConn2 -- Simscape Bus/LConn14
  Tooth Cyl 3/RConn2 -- Simscape Bus/LConn13
  Tooth Cyl 4/RConn2 -- Simscape Bus/LConn12
  Tooth Cyl 5/RConn2 -- Simscape Bus/LConn11

== system sm_ratchet_lifter/Ratchet Lifter/Toothed Rack/left Horiz Cylinders/Tooth Cyl 1 ==
  Cylindrical Solid1 : sm_lib/Body Elements/Cylindrical Solid  GraphicAmbientColor=[0.15 0.15 0.15 1.0]  BasedOnType=Density  CenterOfMass=[0 0 0]  CenterOfMassUnits=m  GraphicDiffuseColor=color.horiz_tooth_cyl_color  CylinderLength=rack.horiz_tooth_cyl_length  CylinderLengthUnits=cm  CylinderRadius=rack.tooth_cyl_rad  CylinderRadiusUnits=cm  Density=1000  DensityUnits=kg/m^3  DoExposeReferenceFrame=on  GraphicEmissiveColor=[0.0 0.0 0.0 1.0]  ExportEntireGeometry=on  SerializedFrames=<Frames/>  MarkerShape=Sphere  MarkerSize=10  GraphicType=FromGeometry  InertiaType=CalculateFromGeometry  Mass=1  MassUnits=kg  MomentsOfInertia=[1 1 1]  MomentsOfInertiaUnits=kg*m^2  GraphicOpacity=1.0  ProductsOfInertia=[0 0 0]  ProductsOfInertiaUnits=kg*m^2  GraphicShininess=75  GraphicSpecularColor=[0.5 0.5 0.5 1.0]  GraphicVisPropType=SimpleVisualProperties
      settings: SourceProductName=Multibody
  Rigid Transform1 : sm_lib/Frames and Transforms/Rigid Transform  TranslationMethod=Cartesian  TranslationStandardOffset=0  TranslationLengthUnit=cm  TranslationStandardAxis=+Z  TranslationCartesianOffset=rack.horiz_tooth_centers(idx, :)  TranslationROffset=0  TranslationROffsetUnits=m  TranslationZOffset=0  TranslationZOffsetUnits=m  TranslationThetaOffset=0  TranslationThetaOffsetUnits=deg  RotationMethod=AlignedAxes  RotationAngleUnits=deg  RotationStandardAxis=+Z  RotationAngle=0.0  RotationArbitraryAxis=[0 0 1]  FollAlignAxisA=+Z  BaseAlignAxisA=+X  FollAlignAxisB=+X  BaseAlignAxisB=+Z  RotationSequenceAxes=FollowerAxes  RotationSequence=XYX  RotationSequenceAngles=[0 0 0]  RotationSequenceAnglesUnits=deg  RotationMatrix=[1 0 0; 0 1 0; 0 0 1]
      settings: SourceProductName=Multibody
  rack : PMIOPort  Side=Right
  G : PMIOPort  Port=2  Side=Right
  connections:
  Cylindrical Solid1/LConn1 -- G/RConn1
  Rigid Transform1/RConn1 -- Cylindrical Solid1/RConn1
  rack/RConn1 -- Rigid Transform1/LConn1

== system sm_ratchet_lifter/Ratchet Lifter/Toothed Rack/left Horiz Cylinders/Tooth Cyl 10 ==
  Cylindrical Solid1 : sm_lib/Body Elements/Cylindrical Solid  GraphicAmbientColor=[0.15 0.15 0.15 1.0]  BasedOnType=Density  CenterOfMass=[0 0 0]  CenterOfMassUnits=m  GraphicDiffuseColor=color.horiz_tooth_cyl_color  CylinderLength=rack.horiz_tooth_cyl_length  CylinderLengthUnits=cm  CylinderRadius=rack.tooth_cyl_rad  CylinderRadiusUnits=cm  Density=1000  DensityUnits=kg/m^3  DoExposeReferenceFrame=on  GraphicEmissiveColor=[0.0 0.0 0.0 1.0]  ExportEntireGeometry=on  SerializedFrames=<Frames/>  MarkerShape=Sphere  MarkerSize=10  GraphicType=FromGeometry  InertiaType=CalculateFromGeometry  Mass=1  MassUnits=kg  MomentsOfInertia=[1 1 1]  MomentsOfInertiaUnits=kg*m^2  GraphicOpacity=1.0  ProductsOfInertia=[0 0 0]  ProductsOfInertiaUnits=kg*m^2  GraphicShininess=75  GraphicSpecularColor=[0.5 0.5 0.5 1.0]  GraphicVisPropType=SimpleVisualProperties
      settings: SourceProductName=Multibody
  Rigid Transform1 : sm_lib/Frames and Transforms/Rigid Transform  TranslationMethod=Cartesian  TranslationStandardOffset=0  TranslationLengthUnit=cm  TranslationStandardAxis=+Z  TranslationCartesianOffset=rack.horiz_tooth_centers(idx, :)  TranslationROffset=0  TranslationROffsetUnits=m  TranslationZOffset=0  TranslationZOffsetUnits=m  TranslationThetaOffset=0  TranslationThetaOffsetUnits=deg  RotationMethod=AlignedAxes  RotationAngleUnits=deg  RotationStandardAxis=+Z  RotationAngle=0.0  RotationArbitraryAxis=[0 0 1]  FollAlignAxisA=+Z  BaseAlignAxisA=+X  FollAlignAxisB=+X  BaseAlignAxisB=+Z  RotationSequenceAxes=FollowerAxes  RotationSequence=XYX  RotationSequenceAngles=[0 0 0]  RotationSequenceAnglesUnits=deg  RotationMatrix=[1 0 0; 0 1 0; 0 0 1]
      settings: SourceProductName=Multibody
  rack : PMIOPort  Side=Right
  G : PMIOPort  Port=2  Side=Right
  connections:
  Cylindrical Solid1/LConn1 -- G/RConn1
  Rigid Transform1/RConn1 -- Cylindrical Solid1/RConn1
  rack/RConn1 -- Rigid Transform1/LConn1

== system sm_ratchet_lifter/Ratchet Lifter/Toothed Rack/left Horiz Cylinders/Tooth Cyl 11 ==
  Cylindrical Solid1 : sm_lib/Body Elements/Cylindrical Solid  GraphicAmbientColor=[0.15 0.15 0.15 1.0]  BasedOnType=Density  CenterOfMass=[0 0 0]  CenterOfMassUnits=m  GraphicDiffuseColor=color.horiz_tooth_cyl_color  CylinderLength=rack.horiz_tooth_cyl_length  CylinderLengthUnits=cm  CylinderRadius=rack.tooth_cyl_rad  CylinderRadiusUnits=cm  Density=1000  DensityUnits=kg/m^3  DoExposeReferenceFrame=on  GraphicEmissiveColor=[0.0 0.0 0.0 1.0]  ExportEntireGeometry=on  SerializedFrames=<Frames/>  MarkerShape=Sphere  MarkerSize=10  GraphicType=FromGeometry  InertiaType=CalculateFromGeometry  Mass=1  MassUnits=kg  MomentsOfInertia=[1 1 1]  MomentsOfInertiaUnits=kg*m^2  GraphicOpacity=1.0  ProductsOfInertia=[0 0 0]  ProductsOfInertiaUnits=kg*m^2  GraphicShininess=75  GraphicSpecularColor=[0.5 0.5 0.5 1.0]  GraphicVisPropType=SimpleVisualProperties
      settings: SourceProductName=Multibody
  Rigid Transform1 : sm_lib/Frames and Transforms/Rigid Transform  TranslationMethod=Cartesian  TranslationStandardOffset=0  TranslationLengthUnit=cm  TranslationStandardAxis=+Z  TranslationCartesianOffset=rack.horiz_tooth_centers(idx, :)  TranslationROffset=0  TranslationROffsetUnits=m  TranslationZOffset=0  TranslationZOffsetUnits=m  TranslationThetaOffset=0  TranslationThetaOffsetUnits=deg  RotationMethod=AlignedAxes  RotationAngleUnits=deg  RotationStandardAxis=+Z  RotationAngle=0.0  RotationArbitraryAxis=[0 0 1]  FollAlignAxisA=+Z  BaseAlignAxisA=+X  FollAlignAxisB=+X  BaseAlignAxisB=+Z  RotationSequenceAxes=FollowerAxes  RotationSequence=XYX  RotationSequenceAngles=[0 0 0]  RotationSequenceAnglesUnits=deg  RotationMatrix=[1 0 0; 0 1 0; 0 0 1]
      settings: SourceProductName=Multibody
  rack : PMIOPort  Side=Right
  G : PMIOPort  Port=2  Side=Right
  connections:
  Cylindrical Solid1/LConn1 -- G/RConn1
  Rigid Transform1/RConn1 -- Cylindrical Solid1/RConn1
  rack/RConn1 -- Rigid Transform1/LConn1

== system sm_ratchet_lifter/Ratchet Lifter/Toothed Rack/left Horiz Cylinders/Tooth Cyl 12 ==
  Cylindrical Solid1 : sm_lib/Body Elements/Cylindrical Solid  GraphicAmbientColor=[0.15 0.15 0.15 1.0]  BasedOnType=Density  CenterOfMass=[0 0 0]  CenterOfMassUnits=m  GraphicDiffuseColor=color.horiz_tooth_cyl_color  CylinderLength=rack.horiz_tooth_cyl_length  CylinderLengthUnits=cm  CylinderRadius=rack.tooth_cyl_rad  CylinderRadiusUnits=cm  Density=1000  DensityUnits=kg/m^3  DoExposeReferenceFrame=on  GraphicEmissiveColor=[0.0 0.0 0.0 1.0]  ExportEntireGeometry=on  SerializedFrames=<Frames/>  MarkerShape=Sphere  MarkerSize=10  GraphicType=FromGeometry  InertiaType=CalculateFromGeometry  Mass=1  MassUnits=kg  MomentsOfInertia=[1 1 1]  MomentsOfInertiaUnits=kg*m^2  GraphicOpacity=1.0  ProductsOfInertia=[0 0 0]  ProductsOfInertiaUnits=kg*m^2  GraphicShininess=75  GraphicSpecularColor=[0.5 0.5 0.5 1.0]  GraphicVisPropType=SimpleVisualProperties
      settings: SourceProductName=Multibody
  Rigid Transform1 : sm_lib/Frames and Transforms/Rigid Transform  TranslationMethod=Cartesian  TranslationStandardOffset=0  TranslationLengthUnit=cm  TranslationStandardAxis=+Z  TranslationCartesianOffset=rack.horiz_tooth_centers(idx, :)  TranslationROffset=0  TranslationROffsetUnits=m  TranslationZOffset=0  TranslationZOffsetUnits=m  TranslationThetaOffset=0  TranslationThetaOffsetUnits=deg  RotationMethod=AlignedAxes  RotationAngleUnits=deg  RotationStandardAxis=+Z  RotationAngle=0.0  RotationArbitraryAxis=[0 0 1]  FollAlignAxisA=+Z  BaseAlignAxisA=+X  FollAlignAxisB=+X  BaseAlignAxisB=+Z  RotationSequenceAxes=FollowerAxes  RotationSequence=XYX  RotationSequenceAngles=[0 0 0]  RotationSequenceAnglesUnits=deg  RotationMatrix=[1 0 0; 0 1 0; 0 0 1]
      settings: SourceProductName=Multibody
  rack : PMIOPort  Side=Right
  G : PMIOPort  Port=2  Side=Right
  connections:
  Cylindrical Solid1/LConn1 -- G/RConn1
  Rigid Transform1/RConn1 -- Cylindrical Solid1/RConn1
  rack/RConn1 -- Rigid Transform1/LConn1

== system sm_ratchet_lifter/Ratchet Lifter/Toothed Rack/left Horiz Cylinders/Tooth Cyl 13 ==
  Cylindrical Solid1 : sm_lib/Body Elements/Cylindrical Solid  GraphicAmbientColor=[0.15 0.15 0.15 1.0]  BasedOnType=Density  CenterOfMass=[0 0 0]  CenterOfMassUnits=m  GraphicDiffuseColor=color.horiz_tooth_cyl_color  CylinderLength=rack.horiz_tooth_cyl_length  CylinderLengthUnits=cm  CylinderRadius=rack.tooth_cyl_rad  CylinderRadiusUnits=cm  Density=1000  DensityUnits=kg/m^3  DoExposeReferenceFrame=on  GraphicEmissiveColor=[0.0 0.0 0.0 1.0]  ExportEntireGeometry=on  SerializedFrames=<Frames/>  MarkerShape=Sphere  MarkerSize=10  GraphicType=FromGeometry  InertiaType=CalculateFromGeometry  Mass=1  MassUnits=kg  MomentsOfInertia=[1 1 1]  MomentsOfInertiaUnits=kg*m^2  GraphicOpacity=1.0  ProductsOfInertia=[0 0 0]  ProductsOfInertiaUnits=kg*m^2  GraphicShininess=75  GraphicSpecularColor=[0.5 0.5 0.5 1.0]  GraphicVisPropType=SimpleVisualProperties
      settings: SourceProductName=Multibody
  Rigid Transform1 : sm_lib/Frames and Transforms/Rigid Transform  TranslationMethod=Cartesian  TranslationStandardOffset=0  TranslationLengthUnit=cm  TranslationStandardAxis=+Z  TranslationCartesianOffset=rack.horiz_tooth_centers(idx, :)  TranslationROffset=0  TranslationROffsetUnits=m  TranslationZOffset=0  TranslationZOffsetUnits=m  TranslationThetaOffset=0  TranslationThetaOffsetUnits=deg  RotationMethod=AlignedAxes  RotationAngleUnits=deg  RotationStandardAxis=+Z  RotationAngle=0.0  RotationArbitraryAxis=[0 0 1]  FollAlignAxisA=+Z  BaseAlignAxisA=+X  FollAlignAxisB=+X  BaseAlignAxisB=+Z  RotationSequenceAxes=FollowerAxes  RotationSequence=XYX  RotationSequenceAngles=[0 0 0]  RotationSequenceAnglesUnits=deg  RotationMatrix=[1 0 0; 0 1 0; 0 0 1]
      settings: SourceProductName=Multibody
  rack : PMIOPort  Side=Right
  G : PMIOPort  Port=2  Side=Right
  connections:
  Cylindrical Solid1/LConn1 -- G/RConn1
  Rigid Transform1/RConn1 -- Cylindrical Solid1/RConn1
  rack/RConn1 -- Rigid Transform1/LConn1

== system sm_ratchet_lifter/Ratchet Lifter/Toothed Rack/left Horiz Cylinders/Tooth Cyl 14 ==
  Cylindrical Solid1 : sm_lib/Body Elements/Cylindrical Solid  GraphicAmbientColor=[0.15 0.15 0.15 1.0]  BasedOnType=Density  CenterOfMass=[0 0 0]  CenterOfMassUnits=m  GraphicDiffuseColor=color.horiz_tooth_cyl_color  CylinderLength=rack.horiz_tooth_cyl_length  CylinderLengthUnits=cm  CylinderRadius=rack.tooth_cyl_rad  CylinderRadiusUnits=cm  Density=1000  DensityUnits=kg/m^3  DoExposeReferenceFrame=on  GraphicEmissiveColor=[0.0 0.0 0.0 1.0]  ExportEntireGeometry=on  SerializedFrames=<Frames/>  MarkerShape=Sphere  MarkerSize=10  GraphicType=FromGeometry  InertiaType=CalculateFromGeometry  Mass=1  MassUnits=kg  MomentsOfInertia=[1 1 1]  MomentsOfInertiaUnits=kg*m^2  GraphicOpacity=1.0  ProductsOfInertia=[0 0 0]  ProductsOfInertiaUnits=kg*m^2  GraphicShininess=75  GraphicSpecularColor=[0.5 0.5 0.5 1.0]  GraphicVisPropType=SimpleVisualProperties
      settings: SourceProductName=Multibody
  Rigid Transform1 : sm_lib/Frames and Transforms/Rigid Transform  TranslationMethod=Cartesian  TranslationStandardOffset=0  TranslationLengthUnit=cm  TranslationStandardAxis=+Z  TranslationCartesianOffset=rack.horiz_tooth_centers(idx, :)  TranslationROffset=0  TranslationROffsetUnits=m  TranslationZOffset=0  TranslationZOffsetUnits=m  TranslationThetaOffset=0  TranslationThetaOffsetUnits=deg  RotationMethod=AlignedAxes  RotationAngleUnits=deg  RotationStandardAxis=+Z  RotationAngle=0.0  RotationArbitraryAxis=[0 0 1]  FollAlignAxisA=+Z  BaseAlignAxisA=+X  FollAlignAxisB=+X  BaseAlignAxisB=+Z  RotationSequenceAxes=FollowerAxes  RotationSequence=XYX  RotationSequenceAngles=[0 0 0]  RotationSequenceAnglesUnits=deg  RotationMatrix=[1 0 0; 0 1 0; 0 0 1]
      settings: SourceProductName=Multibody
  rack : PMIOPort  Side=Right
  G : PMIOPort  Port=2  Side=Right
  connections:
  Cylindrical Solid1/LConn1 -- G/RConn1
  Rigid Transform1/RConn1 -- Cylindrical Solid1/RConn1
  rack/RConn1 -- Rigid Transform1/LConn1
